simulink model "tm4c1294npdt_onboard_button_led"  (R2013b)
settings: Solver=ode3  SolverMode=SingleTasking  StartTime=0.0  StopTime=inf  FixedStep=0.01  RelTol=1e-3
libraries: tm4c1294npdt x6
settings Model: ExtModeTrigDuration=2  Creator=q365198  LastModifiedBy=q365198
settings OptimizationCC: OptimizeModelRefInitCode=on  LifeSpan=1
settings DebuggingCC: SolverPrmCheckMsg=none
settings HardwareCC: ProdLargestAtomicInteger=Long  ProdLargestAtomicFloat=Double  ProdEndianess=LittleEndian  ProdHWDeviceType=ARM Compatible->ARM Cortex
settings RTWCC: SystemTargetFile=realtime.tlc  GenerateMakefile=off  TemplateMakefile=realtime.tmf  Description=Run on Target Hardware  RTWVerbose=off  ProcessScript=realtime_make_rtw_hook
settings STFCustomTargetCC: TargetLibSuffix=.a  GenerateSampleERTMain=on  ERTCustomFileBanners=on  SupportNonInlinedSFcns=off  SupportVariableSizeSignals=on  MATLABClassNameForMDSCustomization=Simulink.SoftwareTarget.ERTCustomization  GRTInterface=off  SystemTargetFile=realtime.tlc
settings ERTTargetCC: CodeReplacementLibrary=ANSI_C  GenerateSampleERTMain=on  ParMdlRefBuildCompliant=off  CompOptLevelCompliant=off  ConcurrentExecutionCompliant=off  CombineOutputUpdateFcns=off  ERTFirstTimeCompliant=off  SupportContinuousTime=on  SupportVariableSizeSignals=on  ModelStepFunctionPrototypeControlCompliant=off  CPPClassGenCompliant=off  ExtModeTransport=3  ExtModeMexFile=ext_serial_win32_comm  ExtModeMexArgs=0 COM12 115200  InlinedParameterPlacement=NonHierarchical  ERTSrcFileBannerTemplate=realtime_code_template.cgt  ERTHdrFileBannerTemplate=realtime_code_template.cgt  ERTDataSrcFileTemplate=realtime_code_template.cgt  ERTDataHdrFileTemplate=realtime_code_template.cgt  ERTCustomFileTemplate=realtime_file_process.tlc

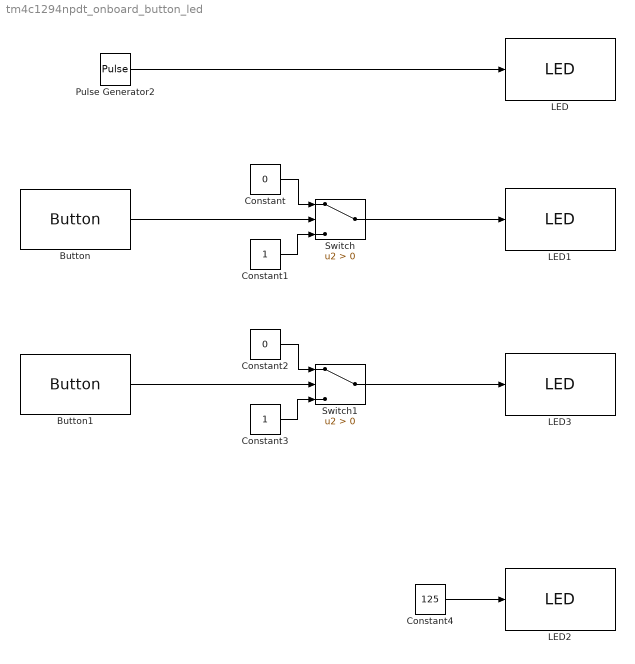
== system tm4c1294npdt_onboard_button_led ==
  Button : tm4c1294npdt/Button  popup_pin=USR_SW1  pin=85  mode_popup=INPUT_PULLUP  mode=3  SampleTime=-1
  Button1 : tm4c1294npdt/Button  popup_pin=USR_SW1  pin=85  mode_popup=INPUT_PULLUP  mode=3  SampleTime=-1
  Constant : Constant  Value=0  OutDataTypeStr=uint8
  Constant1 : Constant  OutDataTypeStr=uint8
  Constant2 : Constant  Value=0  OutDataTypeStr=uint8
  Constant3 : Constant  OutDataTypeStr=uint8
  Constant4 : Constant  Value=125  OutDataTypeStr=uint8
  LED : tm4c1294npdt/LED  popup_led=LED1  pin=81  SampleTime=-1
  LED1 : tm4c1294npdt/LED  popup_led=LED2  pin=82  SampleTime=-1
  LED2 : tm4c1294npdt/LED  popup_led=LED4  pin=84  SampleTime=-1
  LED3 : tm4c1294npdt/LED  popup_led=LED3  pin=83  SampleTime=-1
  Pulse Generator2 : DiscretePulseGenerator  SampleTime=0.05
  Switch : Switch  Criteria=u2 > Threshold
  Switch1 : Switch  Criteria=u2 > Threshold
  wires:
  Pulse Generator2/1 -> LED/1
  Button/1 -> Switch/2
  Constant/1 -> Switch/1
  Constant1/1 -> Switch/3
  Switch/1 -> LED1/1
  Button1/1 -> Switch1/2
  Constant2/1 -> Switch1/1
  Constant3/1 -> Switch1/3
  Constant4/1 -> LED2/1
  Switch1/1 -> LED3/1
